simulink model "ex_modeling_variants"  (R2019b)
settings: Solver=VariableStepAuto  StartTime=0.0  StopTime=30  RelTol=1e-3
PreLoadFcn:
  | addpath(fullfile(matlabroot,'examples','simulink','main'));
  | 
  | ex_modeling_bus_objects
  | ex_modeling_data_mechanical_system
  | ex_modeling_variant_choice
  | 
  | rmpath(fullfile(matlabroot,'examples','simulink','main'));
undefined symbols (not defined in the file): __PRM__SERIALIZED__DATA__, SubsystemReferenceBlock
libraries: simulink x1
settings Model: Creator=The MathWorks, Inc.  LastModifiedBy=The MathWorks, Inc.
settings DataIOCC: ReturnWorkspaceOutputs=off
settings DebuggingCC: ModelReferenceExtraNoncontSigs=warning  PregeneratedLibrarySubsystemCodeDiagnostic=none  ArithmeticOperatorsInVariantConditions=warning
settings SFSimCC: SimUseLocalCustomCode=off  CustomCodeUndefinedFunction=UseInterfaceOnly
settings RTWCC: RTWUseLocalCustomCode=off

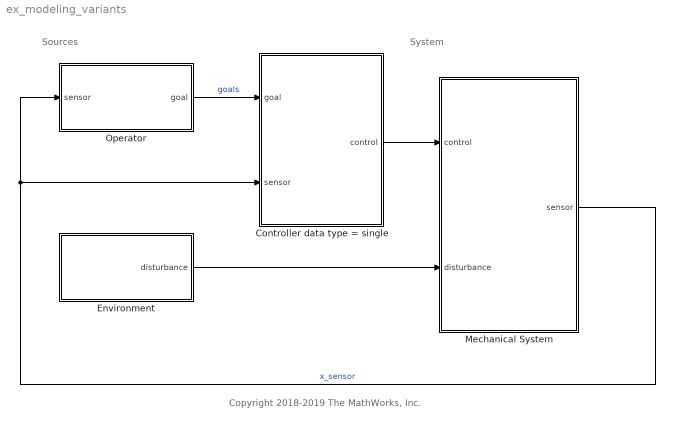
== system ex_modeling_variants ==
  note: System
  note: Sources
  note: Copyright 2018-2019 The MathWorks, Inc.
  Controller data type = single : Subsystem
  Environment : Subsystem
  Mechanical System : Subsystem
  Operator : Subsystem  Variant=on  VariantControl=Variant1
  wires:
  Mechanical System/1(sensor) -> Operator/1(sensor), Controller data type = single/2(sensor)  "x_sensor"
  Environment/1(disturbance) -> Mechanical System/2(disturbance)
  Operator/1(goal) -> Controller data type = single/1(goal)  "goals"
  Controller data type = single/1(control) -> Mechanical System/1(control)

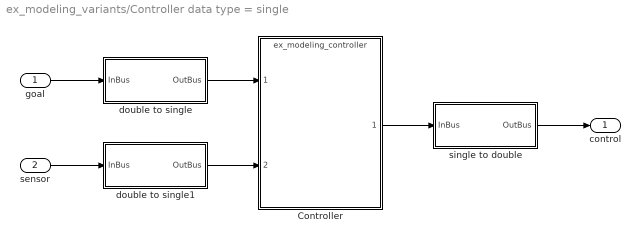
== system ex_modeling_variants/Controller data type = single ==
  goal : Inport
  sensor : Inport  Port=2
  Controller : ModelReference  ModelNameDialog=ex_modeling_controller  SimulationMode=Normal  ModelReferenceVersion=1.71
  double to single : Subsystem
  double to single1 : Subsystem
  single to double : Subsystem
  control : Outport  VectorParamsAs1DForOutWhenUnconnected=off
  wires:
  goal/1 -> double to single/1(InBus)
  sensor/1 -> double to single1/1(InBus)
  Controller/1 -> single to double/1(InBus)
  double to single/1(OutBus) -> Controller/1
  double to single1/1(OutBus) -> Controller/2
  single to double/1(OutBus) -> control/1

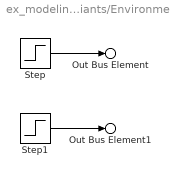
== system ex_modeling_variants/Environment ==
  Step : Step  Time=10  After=10  SampleTime=0
  Step1 : Step  Time=20  After=10  SampleTime=0
  Out Bus Element : Outport  VectorParamsAs1DForOutWhenUnconnected=off  PortName=disturbance  Element=F1
  Out Bus Element1 : Outport  VectorParamsAs1DForOutWhenUnconnected=off  PortName=disturbance  Element=F2
  wires:
  Step/1 -> Out Bus Element/1
  Step1/1 -> Out Bus Element1/1

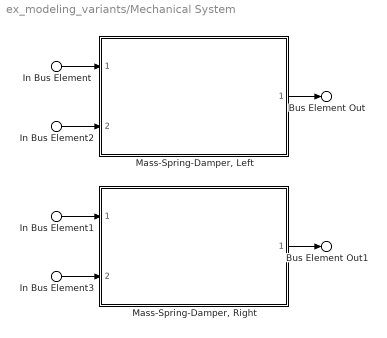
== system ex_modeling_variants/Mechanical System ==
  In Bus Element : Inport  PortName=control  Element=F1
  In Bus Element1 : Inport  PortName=control  Element=F2
  In Bus Element2 : Inport  Port=2  PortName=disturbance  Element=F1
  In Bus Element3 : Inport  Port=2  PortName=disturbance  Element=F2
  "Mass-Spring-Damper, Left" : Subsystem  BlockKeywords=__PRM__SERIALIZED__DATA__:SubsystemReferenceBlock  ReferencedSubsystem=ex_modeling_mechanical_system
  "Mass-Spring-Damper, Right" : Subsystem  BlockKeywords=__PRM__SERIALIZED__DATA__:SubsystemReferenceBlock  ReferencedSubsystem=ex_modeling_mechanical_system
  Bus Element Out : Outport  VectorParamsAs1DForOutWhenUnconnected=off  PortName=sensor  Element=x1
  Bus Element Out1 : Outport  VectorParamsAs1DForOutWhenUnconnected=off  PortName=sensor  Element=x2
  wires:
  In Bus Element2/1 -> "Mass-Spring-Damper, Left"/2
  In Bus Element1/1 -> "Mass-Spring-Damper, Right"/1
  In Bus Element/1 -> "Mass-Spring-Damper, Left"/1
  In Bus Element3/1 -> "Mass-Spring-Damper, Right"/2
  "Mass-Spring-Damper, Right"/1 -> Bus Element Out1/1
  "Mass-Spring-Damper, Left"/1 -> Bus Element Out/1

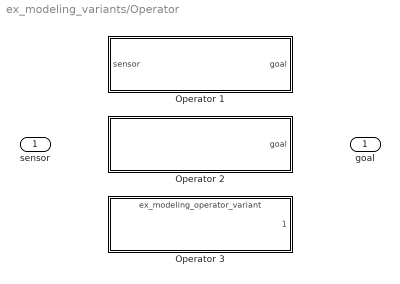
== system ex_modeling_variants/Operator ==
  sensor : Inport
  Operator 1 : Subsystem  VariantControl=operator==1
  Operator 2 : Subsystem  VariantControl=operator==3
  Operator 3 : ModelReference  ModelNameDialog=ex_modeling_operator_variant  SimulationMode=Normal  VariantControl=operator==2  ModelReferenceVersion=1.3
  goal : Outport  VectorParamsAs1DForOutWhenUnconnected=off

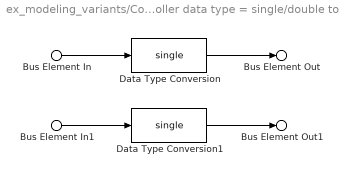
== system ex_modeling_variants/Controller data type = single/double to single ==
  Bus Element In1 : Inport  PortName=InBus  Element=delta_goal
  Bus Element In : Inport  PortName=InBus  Element=x_goal
  Data Type Conversion : DataTypeConversion  OutDataTypeStr=single
  Data Type Conversion1 : DataTypeConversion  OutDataTypeStr=single
  Bus Element Out : Outport  VectorParamsAs1DForOutWhenUnconnected=off  PortName=OutBus  Element=x_goal
  Bus Element Out1 : Outport  VectorParamsAs1DForOutWhenUnconnected=off  PortName=OutBus  Element=delta_goal
  wires:
  Bus Element In/1 -> Data Type Conversion/1
  Data Type Conversion/1 -> Bus Element Out/1
  Data Type Conversion1/1 -> Bus Element Out1/1
  Bus Element In1/1 -> Data Type Conversion1/1

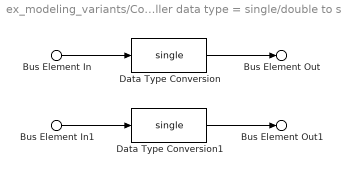
== system ex_modeling_variants/Controller data type = single/double to single1 ==
  Bus Element In1 : Inport  PortName=InBus  Element=x2
  Bus Element In : Inport  PortName=InBus  Element=x1
  Data Type Conversion : DataTypeConversion  OutDataTypeStr=single
  Data Type Conversion1 : DataTypeConversion  OutDataTypeStr=single
  Bus Element Out : Outport  VectorParamsAs1DForOutWhenUnconnected=off  PortName=OutBus  Element=x1
  Bus Element Out1 : Outport  VectorParamsAs1DForOutWhenUnconnected=off  PortName=OutBus  Element=x2
  wires:
  Bus Element In1/1 -> Data Type Conversion1/1
  Data Type Conversion1/1 -> Bus Element Out1/1
  Data Type Conversion/1 -> Bus Element Out/1
  Bus Element In/1 -> Data Type Conversion/1

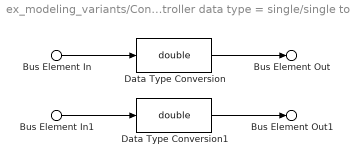
== system ex_modeling_variants/Controller data type = single/single to double ==
  Bus Element In : Inport  PortName=InBus  Element=F1
  Bus Element In1 : Inport  PortName=InBus  Element=F2
  Data Type Conversion : DataTypeConversion  OutDataTypeStr=double
  Data Type Conversion1 : DataTypeConversion  OutDataTypeStr=double
  Bus Element Out : Outport  VectorParamsAs1DForOutWhenUnconnected=off  PortName=OutBus  Element=F1
  Bus Element Out1 : Outport  VectorParamsAs1DForOutWhenUnconnected=off  PortName=OutBus  Element=F2
  wires:
  Bus Element In/1 -> Data Type Conversion/1
  Data Type Conversion/1 -> Bus Element Out/1
  Data Type Conversion1/1 -> Bus Element Out1/1
  Bus Element In1/1 -> Data Type Conversion1/1

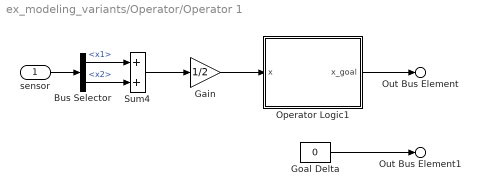
== system ex_modeling_variants/Operator/Operator 1 ==
  sensor : Inport
  Bus Selector : BusSelector  OutputSignals=x1,x2
  Gain : Gain  Gain=1/2
  Goal Delta : Constant  Value=0
  Operator Logic1 : Stateflow chart  TreatAsAtomicUnit=on
  Sum4 : Sum
  Out Bus Element : Outport  VectorParamsAs1DForOutWhenUnconnected=off  PortName=goal  Element=x_goal
  Out Bus Element1 : Outport  VectorParamsAs1DForOutWhenUnconnected=off  PortName=goal  Element=delta_goal
  wires:
  Bus Selector/2 -> Sum4/2  "<x2>"
  Bus Selector/1 -> Sum4/1  "<x1>"
  sensor/1 -> Bus Selector/1
  Operator Logic1/1(x_goal) -> Out Bus Element/1
  Goal Delta/1 -> Out Bus Element1/1
  Sum4/1 -> Gain/1
  Gain/1 -> Operator Logic1/1(x)

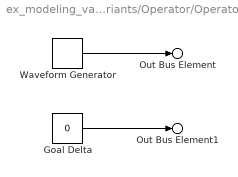
== system ex_modeling_variants/Operator/Operator 2 ==
  Goal Delta : Constant  Value=0
  Waveform Generator : simulink/Sources/Waveform Generator  OutMin=[]  OutMax=[]  OutDataTypeStr=double  SelectedSignal=1  Signals=sin('Amplitude', 0.1, 'Frequency', 10, 'Phase', 1) + step(5,1,2)  BlockNames=MultiportSwitch_3a836cc316f245c  SampleTime=0.01
      settings: SourceProductName=Simulink
  Out Bus Element : Outport  VectorParamsAs1DForOutWhenUnconnected=off  PortName=goal  Element=x_goal
  Out Bus Element1 : Outport  VectorParamsAs1DForOutWhenUnconnected=off  PortName=goal  Element=delta_goal
  wires:
  Waveform Generator/1 -> Out Bus Element/1
  Goal Delta/1 -> Out Bus Element1/1

== stateflow chart ex_modeling_variants/Operator/Operator 1/Operator Logic1 ==
  state wait
    entry: x_goal = 0;
  state FirstOperation
    entry: x_goal = 2;
  state SecondOperation
    entry: x_goal = 1;
  wait -> FirstOperation : after(2,sec)
  FirstOperation -> SecondOperation : [x>2]
  (default) -> wait
  data: x input; x_goal output
